simulink model "omnibot"  (Simulink 8.2)
settings: Solver=ode3  SolverMode=SingleTasking  StartTime=0.0  StopTime=12.0  RelTol=1e-3
libraries: legonxtlib x3, simulink x3
settings Model: Creator=Alphonso Monk  LastModifiedBy=Alphonso Monk  SimulationMode=external  ExtModeTrigDuration=2
settings DataIOCC: SignalLoggingSaveFormat=Dataset
settings OptimizationCC: ExpressionDepthLimit=128  OptimizeModelRefInitCode=on  LifeSpan=1
settings DebuggingCC: SolverPrmCheckMsg=none  FcnCallInpInsideContextMsg=EnableAllAsError  StateNameClashWarn=none
settings HardwareCC: ProdLargestAtomicInteger=Long  ProdLargestAtomicFloat=Float  ProdEndianess=LittleEndian  ProdHWDeviceType=ARM Compatible->ARM 7
settings RTWCC: SystemTargetFile=realtime.tlc  GenerateMakefile=off  TemplateMakefile=realtime.tmf  Description=Run on Target Hardware  RTWVerbose=off  ProcessScript=realtime_make_rtw_hook
settings STFCustomTargetCC: TargetLibSuffix=.a  CodeReplacementLibrary=ANSI_C  GenerateSampleERTMain=on  ERTCustomFileBanners=on  SupportNonInlinedSFcns=off  SupportVariableSizeSignals=on  MATLABClassNameForMDSCustomization=Simulink.SoftwareTarget.ERTCustomization  GRTInterface=off  SystemTargetFile=realtime.tlc
settings ERTTargetCC: CodeReplacementLibrary=ANSI_C  MultiwordLength=2048  GenerateSampleERTMain=on  ParMdlRefBuildCompliant=off  CompOptLevelCompliant=off  ConcurrentExecutionCompliant=off  CombineOutputUpdateFcns=off  ERTFirstTimeCompliant=off  SupportContinuousTime=on  SupportVariableSizeSignals=on  ModelStepFunctionPrototypeControlCompliant=off  CPPClassGenCompliant=off  ExtModeTransport=2  ExtModeMexFile=ext_serial_win32_comm_no_acks_rtt  ExtModeMexArgs=0 1 9600  InlinedParameterPlacement=NonHierarchical  ERTSrcFileBannerTemplate=realtime_code_template.cgt  ERTHdrFileBannerTemplate=realtime_code_template.cgt  ERTDataSrcFileTemplate=realtime_code_template.cgt  ERTDataHdrFileTemplate=realtime_code_template.cgt  ERTCustomFileTemplate=realtime_file_process.tlc  ConvertIfToSwitch=off  SuppressUnreachableDefaultCases=off
settings SettingsController: Description=Run on Hardware Dialog  TargetExtensionPlatform=LEGO MINDSTORMS NXT
settings MATStruct: COM_port_number=1  Find_com_port=[0.0]  Enable_overrun_detection=[0.0]  Enable_LEGO_to_LEGO_communication=[0.0]  Bluetooth_mode=[0.0]  Slave_bluetooth_address=00:16:53:0f:0c:09

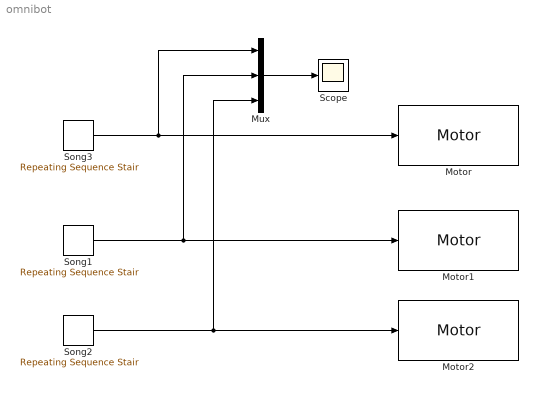
== system omnibot ==
  Motor : legonxtlib/Motor  sportNumber=A  sstopAction=Brake
  Motor1 : legonxtlib/Motor  sportNumber=C  sstopAction=Brake
  Motor2 : legonxtlib/Motor  sportNumber=B  sstopAction=Brake
  Mux : Mux  Inputs=3
  Scope : Scope
  Song1 : simulink/Sources/Repeating Sequence Stair  OutValues=[0 50 -100 0].'  tsamp=2  OutMin=[]  OutMax=[]  OutDataTypeStr=int32  OutputDataTypeScalingMode=int32  OutDataType=fixdt(0,8)  ConRadixGroup=Best Precision: Vector-wise  OutScaling=2^-12
  Song2 : simulink/Sources/Repeating Sequence Stair  OutValues=[100 -50 100 0].'  tsamp=2  OutMin=[]  OutMax=[]  OutDataTypeStr=int32  OutputDataTypeScalingMode=int32  OutDataType=fixdt(0,8)  ConRadixGroup=Best Precision: Vector-wise  OutScaling=2^-12
  Song3 : simulink/Sources/Repeating Sequence Stair  OutValues=[-100 50 100 0].'  tsamp=2  OutMin=[]  OutMax=[]  OutDataTypeStr=int32  OutputDataTypeScalingMode=int32  OutDataType=fixdt(0,8)  ConRadixGroup=Best Precision: Vector-wise  OutScaling=2^-12
  wires:
  Song3/1 -> Mux/1, Motor/1
  Song1/1 -> Mux/2, Motor1/1
  Song2/1 -> Mux/3, Motor2/1
  Mux/1 -> Scope/1
